simulink model "MicroMouseDebug"  (R2023a)
settings: Solver=VariableStepAuto  StartTime=0.0  StopTime=inf  FixedStep=0.001  RelTol=1e-3
model workspace (MAT data in the model file):
  comPort = "COM6"
  numBytes = Simulink.Parameter
  numBytes.Value = 5
  numBytes.DataType = 'auto'
  numBytes.Complexity = 'real'
  numBytes.Dimensions = [1 1]
libraries: etargetslib x37, dspstat3 x34, instrumentseriallib x2, stmutilitieslib x1
settings Model: Creator=JesseJabezArendse  LastModifiedBy=JesseJabezArendse
settings DataIOCC: SaveOutput=off  SaveTime=off
settings OptimizationCC: DefaultParameterBehavior=Inlined  InlineInvariantSignals=on  EnhancedBackFolding=on  PassReuseOutputArgsAs=Individual arguments  StateBitsets=on  DataBitsets=on  ZeroExternalMemoryAtStartup=off  ZeroInternalMemoryAtStartup=off  NoFixptDivByZeroProtection=on  EfficientFloat2IntCast=on  OptimizeBlockOrder=speed  DifferentSizesBufferReuse=on  EfficientTunableParamExpr=on
settings DebuggingCC: ParameterPrecisionLossMsg=none  ParameterTunabilityLossMsg=error
settings SFSimCC: MATLABDynamicMemAlloc=off
settings RTWCC: Description=Embedded Coder  SystemTargetFile=ert.tlc  TemplateMakefile=ert_default_tmf  GenerateReport=on  RTWVerbose=off  IncludeHyperlinkInReport=on  LaunchReport=on  GenerateTraceInfo=on  GenerateTraceReport=on  GenerateTraceReportSl=on  GenerateTraceReportSf=on  GenerateTraceReportEml=on
settings CodeAppCC: ForceParamTrailComments=on  IgnoreCustomStorageClasses=off  OperatorAnnotations=on  SimulinkDataObjDesc=on  SFDataObjDesc=on  CustomSymbolStrGlobalVar=rt$N$M  CustomSymbolStrType=$N$M  CustomSymbolStrFcn=$N$M$F  CustomSymbolStrMacro=$N$M  InsertBlockDesc=on
settings ERTTargetCC: TargetLangStandard=C99 (ISO)  GenerateSampleERTMain=on  IncludeMdlTerminateFcn=off  CombineSignalStateStructs=on  PurelyIntegerCode=on  SupportNonFinite=off  InlinedParameterPlacement=NonHierarchical  ERTCustomFileTemplate=example_file_process.tlc

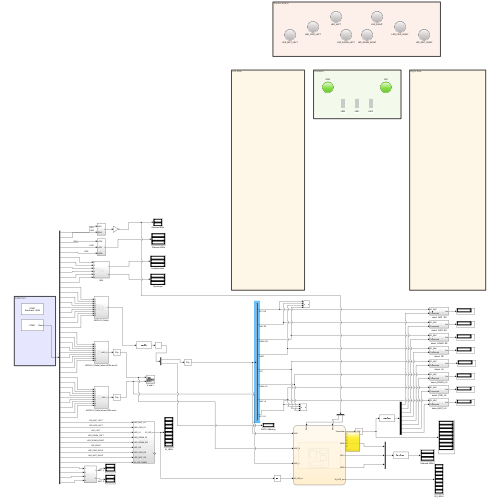
[thumbnail: Simulink's stored preview of the top-level diagram]
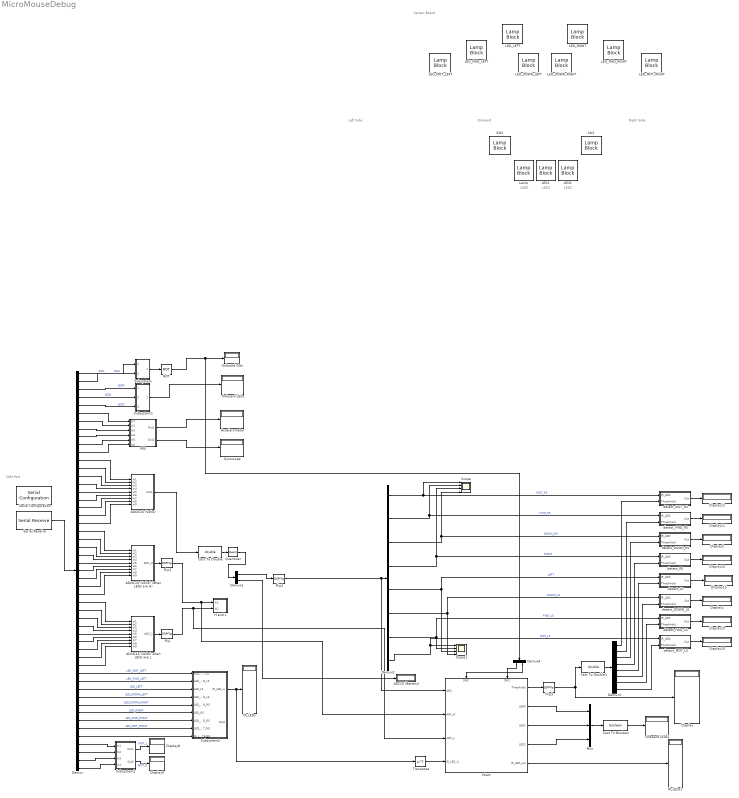
== system MicroMouseDebug ==
  note: Onboard
  note: LED0
  note: LED1
  note: LED2
  note: Left Side
  note: COM Port
  note: Right Side
  note: Sensor Board
  ADC16 (Battery) : Display
  ADC8-16 (Volts) : Subsystem
  ADC8-16 (Volts) (when LEDs are H) : Subsystem
  ADC8-16 (Volts) when LEDs are L : Subsystem
  Accelerometer : Display
  Cast To Boolean : DataTypeConversion  OutDataTypeStr=boolean  SaturateOnIntegerOverflow=off  RndMeth=Floor
  Cast To Double : DataTypeConversion  OutDataTypeStr=double  SaturateOnIntegerOverflow=off  RndMeth=Floor
  Cast To Double1 : DataTypeConversion  OutDataTypeStr=double  SaturateOnIntegerOverflow=off  RndMeth=Floor
  Chart : Stateflow chart  TreatAsAtomicUnit=on
      settings: PortSchema="{\"entries\":[{\"content\":{\"sides\":[{\"content\":{\"connectorIds\":[\"In1\",\"In4\",\"In5\",\"In6\"]},\"type\":\"ConnectorPlacement.EquallySpacedRectSide\",\"uuid\":\"32f6fed0-3232-4bab-b39d-a3af84b75639\"},{\"content\":{\"connectorIds\":[\"Out5\",\"Out1\",\"Out2\",\"Out3\",\"Out4\"],\"side\":\"RIGHT\"},\"type\":\"ConnectorPlacement.EquallySpacedRectSide\",\"uuid\":\"0c32a1fe-915a-4e8a-b3ee-800457e23572\"},{\"content\":{\"connectorIds\":[\"In3\",\"In2\"],\"side\":\"TOP\"},\"type\":\"ConnectorPlacement.EquallySpacedRectSide\",\"uuid\":\"1ac04b60-bb97-4700-a588-8796c93b1b04\"}]},\"type\":\"ConnectorPlacement.EquallySpacedConnector\",\"uuid\":\"e2f36b59-a9e2-4f43-a02a-04bcc2f7ebe2\"}],\"packageUris\":[\"http://schema.mathworks.com/mf0/Connector/R2020b\"],\"version\":\"1.0\"}"
  Demux : Demux  Outputs=[1 1 1 1 1 4 4 4 4 4 4 2 2 2 2 2 2 2 2 2 2 2 2 2 2 2 2 2 2 2 2 2 2 2 2 2 2 2 1 1 1 1 1 1 1 1 4 2 2 2 2]
  Demux1 : Demux  Outputs=[8 1]
  Demux2 : Demux  Outputs=8
  Demux3 : Demux  Outputs=8
  Demux4 : Demux  Outputs=2
  Display{,1..2,8..15} (11 alike) : Display
  Flip{,1..3} (4 alike) : DSPFlip
  Gyroscope : Display
  H and L : Subsystem
  IMU : Subsystem
  IR_LEDs : Display
  IR_LEDs1 : Display
  LED1 : LampBlock  LabelPosition=Hide  Icon=Rectangle
  LED2 : LampBlock  LabelPosition=Hide  Icon=Rectangle
  LED_DOWN_LEFT : LampBlock  LabelPosition=Hide
  LED_DOWN_RIGHT : LampBlock  LabelPosition=Hide
  LED_FWD_LEFT : LampBlock  LabelPosition=Hide
  LED_FWD_RIGHT : LampBlock  LabelPosition=Hide
  LED_LEFT : LampBlock  LabelPosition=Hide
  LED_MOT_LEFT : LampBlock  LabelPosition=Hide
  LED_MOT_RIGHT : LampBlock  LabelPosition=Hide
  LED_RIGHT : LampBlock  LabelPosition=Hide
  Lamp : LampBlock  LabelPosition=Hide  Icon=Rectangle
  Mux : Mux  Inputs=3
  NOT : Logic  Operator=NOT  IconShape=distinctive  AllPortsSameDT=off  OutDataTypeStr=boolean
  Onboard LEDs : Display
  Onboard LEDs1 : Display
  Onboard SWs : Display
  Quantizer : Quantizer  QuantizationInterval=0.01
  SW1 : LampBlock  LabelPosition=Hide
  SW2 : LampBlock  LabelPosition=Hide
  Scope : Scope  NumInputPorts=4
  Scope1 : Scope  NumInputPorts=4
  Serial Configuration : instrumentseriallib/Serial Configuration  Priority=-200000  PortSel=COM7  Port=COM7  ComPort=COM7  BaudRate=9600  DataBits=8  Parity=none  StopBits=1  ByteOrder=little-endian  FlowControl=none  Timeout=10  SimulateUsing=Interpreted execution  BlockInModel=on  aMode=1
      settings: LibrarySourceBlock=embeddedtargetslib/Host Communication/Serial Configuration
  Serial Receive : instrumentseriallib/Serial Receive  Priority=1  PortSel=COM7  Port=COM7  ComPort=COM7  DataType=uint8  SaveDataType=uint8  ToggleHeader=on  Header='JJA'  ToggleTerminator=on  Terminator=Custom terminator  CustomTerminator='3099'  InputFormat=Column major  ToggleDataSize=on  DataSize=[1 103]  EnableBlockingMode=on  ActionDataUnavailable=Output last received value  ActionWhenDataUnavailable=Output last received value  CustomValue=0  SampleTime=0.01  SimulateUsing=Interpreted execution  BlockInModel=on  aMode=1
      settings: LibrarySourceBlock=embeddedtargetslib/Host Communication/Serial Receive
  Subsystem : Subsystem
  Subsystem1 : Subsystem
  Subsystem2 : Subsystem
  Subsystem3 : Subsystem
  Transpose : Math  Operator=transpose
  detect_DOWN_LS : Subsystem
  detect_DOWN_RS : Subsystem
  detect_FWD_LS : Subsystem
  detect_FWD_RS : Subsystem
  detect_LS : Subsystem
  detect_MOT_LS : Subsystem
  detect_MOT_RS : Subsystem
  detect_RS : Subsystem
  wires:
  Serial Receive/1 -> Demux/1
  Demux1/2 -> ADC16 (Battery)/1
  Demux/12 -> ADC8-16 (Volts)/1(In1)
  Demux/13 -> ADC8-16 (Volts)/2(In2)
  Demux/14 -> ADC8-16 (Volts)/3(In3)
  Demux/15 -> ADC8-16 (Volts)/4(In4)
  Demux/16 -> ADC8-16 (Volts)/5(In5)
  Demux/17 -> ADC8-16 (Volts)/6(In6)
  Demux/18 -> ADC8-16 (Volts)/7(In7)
  Demux/19 -> ADC8-16 (Volts)/8(In8)
  Demux/20 -> ADC8-16 (Volts)/9(In9)
  Demux/6 -> IMU/1(In1)
  Demux/7 -> IMU/2(In2)
  Demux/8 -> IMU/3(In3)
  Demux/9 -> IMU/4(In4)
  Demux/10 -> IMU/5(In5)
  Demux/11 -> IMU/6(In6)
  IMU/1(Out1) -> Accelerometer/1
  IMU/2(Out2) -> Gyroscope/1
  Demux/1 -> Subsystem/1(SW1)  "SW1"
  Demux/2 -> Subsystem/2(SW2)  "SW2"
  Subsystem/1(Out1) -> NOT/1
  Demux/3 -> Subsystem1/1(LED0)  "LED0"
  Demux/4 -> Subsystem1/2(LED1)  "LED1"
  Demux/5 -> Subsystem1/3(LED2)  "LED2"
  Subsystem1/1(Out1) -> Onboard LEDs/1
  Demux/38 -> ADC8-16 (Volts) when LEDs are L/9(In9)
  Demux/37 -> ADC8-16 (Volts) when LEDs are L/8(In8)
  Demux/34 -> ADC8-16 (Volts) when LEDs are L/5(In5)
  Demux/33 -> ADC8-16 (Volts) when LEDs are L/4(In4)
  Demux/35 -> ADC8-16 (Volts) when LEDs are L/6(In6)
  Demux/32 -> ADC8-16 (Volts) when LEDs are L/3(In3)
  Demux/36 -> ADC8-16 (Volts) when LEDs are L/7(In7)
  Demux/31 -> ADC8-16 (Volts) when LEDs are L/2(In2)
  Demux/30 -> ADC8-16 (Volts) when LEDs are L/1(In1)
  Demux/29 -> ADC8-16 (Volts) (when LEDs are H)/9(In9)
  Demux/28 -> ADC8-16 (Volts) (when LEDs are H)/8(In8)
  Demux/25 -> ADC8-16 (Volts) (when LEDs are H)/5(In5)
  Demux/24 -> ADC8-16 (Volts) (when LEDs are H)/4(In4)
  Demux/26 -> ADC8-16 (Volts) (when LEDs are H)/6(In6)
  Demux/23 -> ADC8-16 (Volts) (when LEDs are H)/3(In3)
  Demux/27 -> ADC8-16 (Volts) (when LEDs are H)/7(In7)
  Demux/22 -> ADC8-16 (Volts) (when LEDs are H)/2(In2)
  Demux/21 -> ADC8-16 (Volts) (when LEDs are H)/1(In1)
  Demux/39 -> Subsystem3/1(LED_MOT_LS)  "LED_MOT_LEFT"
  Demux/40 -> Subsystem3/2(LED_FWD_LS)  "LED_FWD_LEFT"
  Demux/41 -> Subsystem3/3(LED_LS)  "LED_LEFT"
  Demux/46 -> Subsystem3/8(LED_MOT_RS)  "LED_MOT_RIGHT"
  Demux/47 -> Subsystem3/9(IR_LED_TIMER)
  ADC8-16 (Volts)/1(Out1) -> Cast To Double/1
  detect_FWD_LS/1(Out) -> Display13/1
  Cast To Double/1 -> Quantizer/1
  detect_MOT_LS/1(Out) -> Display10/1
  detect_FWD_RS/1(Out) -> Display11/1
  detect_MOT_RS/1(Out) -> Display12/1
  detect_RS/1(Out) -> Display14/1
  detect_LS/1(Out) -> Display15/1
  Subsystem2/2(Out2) -> Display9/1  "MOT_R"
  Demux/50 -> Subsystem2/3(In3)
  Demux/48 -> Subsystem2/1(In1)
  Demux/51 -> Subsystem2/4(In4)
  Subsystem2/1(Out1) -> Display8/1  "MOT_L"
  Demux/49 -> Subsystem2/2(In2)
  Demux/42 -> Subsystem3/4(LED_DOWN_LS)  "LED_DOWN_LEFT"
  Demux/43 -> Subsystem3/5(LED_DOWN_RS)  "LED_DOWN_RIGHT"
  Demux/44 -> Subsystem3/6(LED_RS)  "LED_RIGHT"
  Demux/45 -> Subsystem3/7(LED_FWD_RS)  "LED_FWD_RIGHT"
  Demux2/1 -> detect_MOT_RS/1(IR_ADC), Scope/1  "MOT_RS"
  Demux2/2 -> Scope/2, detect_FWD_RS/1(IR_ADC)  "FWD_RS"
  Demux2/3 -> Scope/4, detect_DOWN_RS/1(IR_ADC)  "DOWN_RS"
  Demux2/4 -> Scope/3, detect_RS/1(IR_ADC)  "RIGHT"
  Demux2/5 -> detect_LS/1(IR_ADC), Scope1/3  "LEFT"
  Demux2/6 -> detect_DOWN_LS/1(IR_ADC), Scope1/4  "DOWN_LS"
  Demux2/7 -> detect_FWD_LS/1(IR_ADC), Scope1/2  "FWD_LS"
  Demux2/8 -> detect_MOT_LS/1(IR_ADC), Scope1/1  "MOT_LS"
  detect_DOWN_LS/1(Out) -> Display1/1
  detect_DOWN_RS/1(Out) -> Display2/1
  Quantizer/1 -> Demux1/1
  Subsystem3/1(IR_LED_in) -> Transpose/1, IR_LEDs/1
  Chart/1(LED0) -> Mux/1
  Chart/2(LED1) -> Mux/2
  Chart/3(LED2) -> Mux/3
  Mux/1 -> Cast To Boolean/1
  Demux1/1 -> Flip2/1
  ADC8-16 (Volts) (when LEDs are H)/1(ADC_H) -> Flip1/1
  ADC8-16 (Volts) when LEDs are L/1(ADC_L) -> Flip/1
  Chart/4(IR_LED_out) -> IR_LEDs1/1
  Chart/5(Thresholds) -> Flip3/1
  Flip/1 -> Chart/5(ADC_L), H and L/2(In2)
  Flip1/1 -> Chart/4(ADC_H), H and L/1(In1)
  Flip2/1 -> Chart/1(ADC), Demux2/1
  Demux3/1 -> detect_MOT_RS/2(Threshhold)
  Demux3/2 -> detect_FWD_RS/2(Threshhold)
  Demux3/3 -> detect_DOWN_RS/2(Threshhold)
  Demux3/4 -> detect_RS/2(Threshhold)
  Demux3/5 -> detect_LS/2(Threshhold)
  Demux3/6 -> detect_DOWN_LS/2(Threshhold)
  Demux3/7 -> detect_FWD_LS/2(Threshhold)
  Demux3/8 -> detect_MOT_LS/2(Threshhold)
  Demux4/1 -> Chart/2(SW1)
  Demux4/2 -> Chart/3(SW2)
  Transpose/1 -> Chart/6(IR_LED_in)
  Cast To Boolean/1 -> Onboard LEDs1/1
  Cast To Double1/1 -> Demux3/1
  NOT/1 -> Demux4/1, Onboard SWs/1
  Flip3/1 -> Display/1, Cast To Double1/1

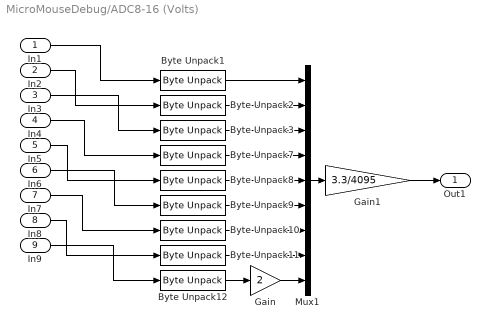
== system MicroMouseDebug/ADC8-16 (Volts) ==
  In1 : Inport
  In2 : Inport  Port=2
  In3 : Inport  Port=3
  In4 : Inport  Port=4
  In5 : Inport  Port=5
  In6 : Inport  Port=6
  In7 : Inport  Port=7
  In8 : Inport  Port=8
  In9 : Inport  Port=9
  Byte Unpack{1..3,7..12} (9 alike) : etargetslib/Byte Unpack  dimensions={[1]}  datatypes={'uint16'}  byteAlign=1
  Gain : Gain  Gain=2  OutDataTypeStr=uint16
  Gain1 : Gain  Gain=3.3/4095
  Mux1 : Mux  Inputs=9
  Out1 : Outport
  wires:
  In7/1 -> Byte Unpack10/1
  Byte Unpack11/1 -> Mux1/8
  Byte Unpack8/1 -> Mux1/5
  Byte Unpack2/1 -> Mux1/2
  Byte Unpack12/1 -> Gain/1
  Byte Unpack7/1 -> Mux1/4
  In4/1 -> Byte Unpack7/1
  Byte Unpack1/1 -> Mux1/1
  In1/1 -> Byte Unpack1/1
  Gain/1 -> Mux1/9
  In6/1 -> Byte Unpack9/1
  Byte Unpack10/1 -> Mux1/7
  Byte Unpack9/1 -> Mux1/6
  Byte Unpack3/1 -> Mux1/3
  Mux1/1 -> Gain1/1
  Gain1/1 -> Out1/1
  In8/1 -> Byte Unpack11/1
  In3/1 -> Byte Unpack3/1
  In5/1 -> Byte Unpack8/1
  In2/1 -> Byte Unpack2/1
  In9/1 -> Byte Unpack12/1

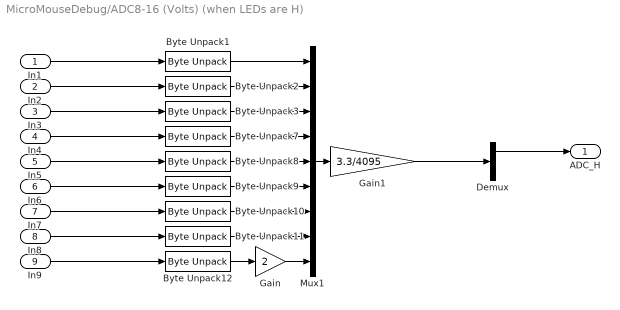
== system MicroMouseDebug/ADC8-16 (Volts) (when LEDs are H) ==
  In1 : Inport
  In2 : Inport  Port=2
  In3 : Inport  Port=3
  In4 : Inport  Port=4
  In5 : Inport  Port=5
  In6 : Inport  Port=6
  In7 : Inport  Port=7
  In8 : Inport  Port=8
  In9 : Inport  Port=9
  Byte Unpack{1..3,7..12} (9 alike) : etargetslib/Byte Unpack  dimensions={[1]}  datatypes={'uint16'}  byteAlign=1
  Demux : Demux  Outputs=[8 1]
  Gain : Gain  Gain=2  OutDataTypeStr=uint16
  Gain1 : Gain  Gain=3.3/4095
  Mux1 : Mux  Inputs=9
  ADC_H : Outport
  wires:
  In7/1 -> Byte Unpack10/1
  Byte Unpack11/1 -> Mux1/8
  Byte Unpack8/1 -> Mux1/5
  Byte Unpack2/1 -> Mux1/2
  Byte Unpack12/1 -> Gain/1
  Byte Unpack7/1 -> Mux1/4
  In4/1 -> Byte Unpack7/1
  Byte Unpack1/1 -> Mux1/1
  In1/1 -> Byte Unpack1/1
  Gain/1 -> Mux1/9
  In6/1 -> Byte Unpack9/1
  Byte Unpack10/1 -> Mux1/7
  Byte Unpack9/1 -> Mux1/6
  Byte Unpack3/1 -> Mux1/3
  Mux1/1 -> Gain1/1
  Gain1/1 -> Demux/1
  In8/1 -> Byte Unpack11/1
  In3/1 -> Byte Unpack3/1
  In5/1 -> Byte Unpack8/1
  In2/1 -> Byte Unpack2/1
  In9/1 -> Byte Unpack12/1
  Demux/1 -> ADC_H/1

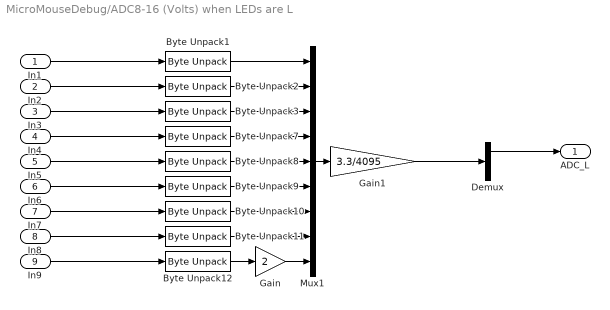
== system MicroMouseDebug/ADC8-16 (Volts) when LEDs are L ==
  In1 : Inport
  In2 : Inport  Port=2
  In3 : Inport  Port=3
  In4 : Inport  Port=4
  In5 : Inport  Port=5
  In6 : Inport  Port=6
  In7 : Inport  Port=7
  In8 : Inport  Port=8
  In9 : Inport  Port=9
  Byte Unpack{1..3,7..12} (9 alike) : etargetslib/Byte Unpack  dimensions={[1]}  datatypes={'uint16'}  byteAlign=1
  Demux : Demux  Outputs=[8 1]
  Gain : Gain  Gain=2  OutDataTypeStr=uint16
  Gain1 : Gain  Gain=3.3/4095
  Mux1 : Mux  Inputs=9
  ADC_L : Outport
  wires:
  In7/1 -> Byte Unpack10/1
  Byte Unpack11/1 -> Mux1/8
  Byte Unpack8/1 -> Mux1/5
  Byte Unpack2/1 -> Mux1/2
  Byte Unpack12/1 -> Gain/1
  Byte Unpack7/1 -> Mux1/4
  In4/1 -> Byte Unpack7/1
  Byte Unpack1/1 -> Mux1/1
  In1/1 -> Byte Unpack1/1
  Gain/1 -> Mux1/9
  In6/1 -> Byte Unpack9/1
  Byte Unpack10/1 -> Mux1/7
  Byte Unpack9/1 -> Mux1/6
  Byte Unpack3/1 -> Mux1/3
  Mux1/1 -> Gain1/1
  In8/1 -> Byte Unpack11/1
  In3/1 -> Byte Unpack3/1
  In5/1 -> Byte Unpack8/1
  In2/1 -> Byte Unpack2/1
  In9/1 -> Byte Unpack12/1
  Gain1/1 -> Demux/1
  Demux/1 -> ADC_L/1

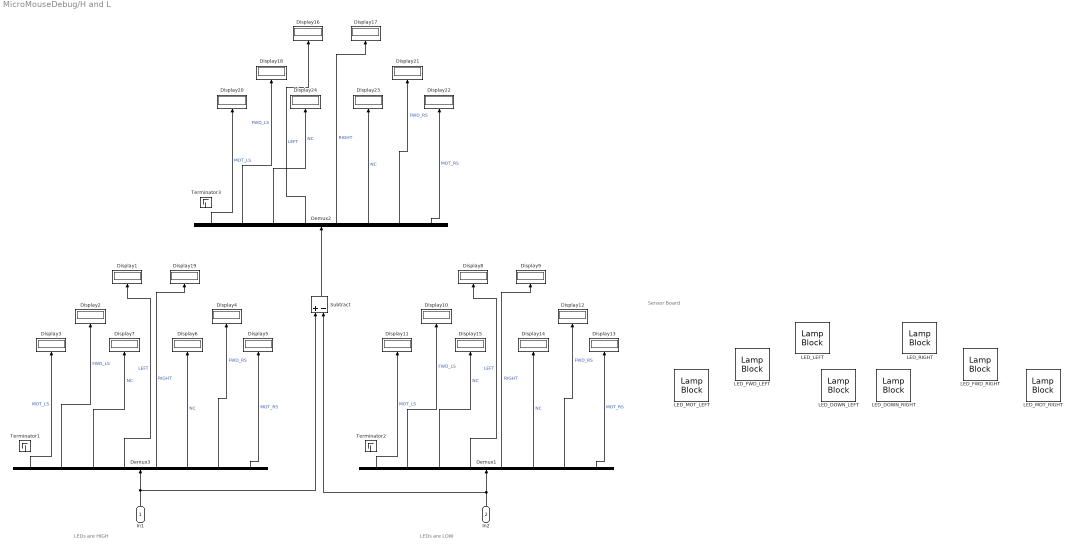
== system MicroMouseDebug/H and L ==
  note: LEDs are HIGH
  note: Sensor Board
  note: LEDs are LOW
  In1 : Inport
  In2 : Inport  Port=2
  Demux1 : Demux  Outputs=8
  Demux2 : Demux  Outputs=8
  Demux3 : Demux  Outputs=8
  Display{1..24} (24 alike) : Display
      settings: Decimation=2
  LED_DOWN_LEFT : LampBlock  LabelPosition=Hide
  LED_DOWN_RIGHT : LampBlock  LabelPosition=Hide
  LED_FWD_LEFT : LampBlock  LabelPosition=Hide
  LED_FWD_RIGHT : LampBlock  LabelPosition=Hide
  LED_LEFT : LampBlock  LabelPosition=Hide
  LED_MOT_LEFT : LampBlock  LabelPosition=Hide
  LED_MOT_RIGHT : LampBlock  LabelPosition=Hide
  LED_RIGHT : LampBlock  LabelPosition=Hide
  Subtract : Sum  Inputs=+-  AccumDataTypeStr=double  OutDataTypeStr=Inherit: Same as accumulator  RndMeth=Nearest  SaturateOnIntegerOverflow=on
  Terminator1 : Terminator
  Terminator2 : Terminator
  Terminator3 : Terminator
  wires:
  Demux3/5 -> Display1/1  "LEFT"
  Demux3/2 -> Display4/1  "FWD_RS"
  Demux3/7 -> Display2/1  "FWD_LS"
  Demux3/4 -> Display19/1  "RIGHT"
  Demux3/8 -> Display3/1  "MOT_LS"
  Demux3/3 -> Display6/1  "NC"
  Demux3/6 -> Display7/1  "NC"
  Demux3/1 -> Display5/1  "MOT_RS"
  ? -> Terminator1/1
  In1/1 -> Demux3/1, Subtract/1
  Demux1/2 -> Display12/1  "FWD_RS"
  In2/1 -> Demux1/1, Subtract/2
  Demux1/1 -> Display13/1  "MOT_RS"
  Demux1/3 -> Display14/1  "NC"
  Demux1/5 -> Display8/1  "LEFT"
  Demux1/8 -> Display11/1  "MOT_LS"
  Demux1/4 -> Display9/1  "RIGHT"
  Demux1/6 -> Display15/1  "NC"
  ? -> Terminator2/1
  Demux1/7 -> Display10/1  "FWD_LS"
  Demux2/2 -> Display21/1  "FWD_RS"
  Demux2/1 -> Display22/1  "MOT_RS"
  Demux2/3 -> Display23/1  "NC"
  Demux2/5 -> Display16/1  "LEFT"
  Demux2/8 -> Display20/1  "MOT_LS"
  Demux2/4 -> Display17/1  "RIGHT"
  Demux2/6 -> Display24/1  "NC"
  ? -> Terminator3/1
  Demux2/7 -> Display18/1  "FWD_LS"
  Subtract/1 -> Demux2/1

== system MicroMouseDebug/IMU ==
  In1 : Inport
  In2 : Inport  Port=2
  In3 : Inport  Port=3
  In4 : Inport  Port=4
  In5 : Inport  Port=5
  In6 : Inport  Port=6
  Byte Unpack{4..6,13..15} (6 alike) : etargetslib/Byte Unpack  dimensions={[1]}  datatypes={'single'}  byteAlign=1
  Mux : Mux  Inputs=3
  Mux2 : Mux  Inputs=3
  Out1 : Outport
  Out2 : Outport  Port=2
  wires:
  Byte Unpack4/1 -> Mux/1
  Byte Unpack14/1 -> Mux2/2
  Byte Unpack15/1 -> Mux2/3
  Mux2/1 -> Out2/1
  Byte Unpack13/1 -> Mux2/1
  In6/1 -> Byte Unpack15/1
  In3/1 -> Byte Unpack6/1
  Byte Unpack5/1 -> Mux/2
  Byte Unpack6/1 -> Mux/3
  In4/1 -> Byte Unpack13/1
  In1/1 -> Byte Unpack4/1
  In2/1 -> Byte Unpack5/1
  Mux/1 -> Out1/1
  In5/1 -> Byte Unpack14/1

== system MicroMouseDebug/Subsystem ==
  SW1 : Inport
  SW2 : Inport  Port=2
  Mux4 : Mux  Inputs=2
  Out1 : Outport
  wires:
  Mux4/1 -> Out1/1
  SW2/1 -> Mux4/2
  SW1/1 -> Mux4/1

== system MicroMouseDebug/Subsystem1 ==
  LED0 : Inport
  LED1 : Inport  Port=2
  LED2 : Inport  Port=3
  Mux3 : Mux  Inputs=3
  Out1 : Outport
  wires:
  Mux3/1 -> Out1/1
  LED2/1 -> Mux3/3
  LED0/1 -> Mux3/1
  LED1/1 -> Mux3/2

== system MicroMouseDebug/Subsystem2 ==
  In1 : Inport
  In2 : Inport  Port=2
  In3 : Inport  Port=3
  In4 : Inport  Port=4
  Byte Unpack{1..3,7} (4 alike) : etargetslib/Byte Unpack  dimensions={[1]}  datatypes={'uint16'}  byteAlign=1
  Gain : Gain  Gain=100/1600
  Gain1 : Gain  Gain=100/1600
  Mux1 : Mux  Inputs=2
  Mux2 : Mux  Inputs=2
  Out1 : Outport
  Out2 : Outport  Port=2
  wires:
  Byte Unpack2/1 -> Mux1/2  "MOT_L_BWD"
  In1/1 -> Byte Unpack1/1
  Byte Unpack3/1 -> Mux2/1  "MOT_R_FWD"
  Mux2/1 -> Gain1/1
  Byte Unpack7/1 -> Mux2/2  "MOT_R_BWD"
  Mux1/1 -> Gain/1
  Gain/1 -> Out1/1
  Byte Unpack1/1 -> Mux1/1  "MOT_L_FWD"
  In3/1 -> Byte Unpack3/1
  In2/1 -> Byte Unpack2/1
  In4/1 -> Byte Unpack7/1
  Gain1/1 -> Out2/1

== system MicroMouseDebug/Subsystem3 ==
  LED_MOT_LS : Inport
  LED_FWD_LS : Inport  Port=2
  LED_LS : Inport  Port=3
  LED_DOWN_LS : Inport  Port=4
  LED_DOWN_RS : Inport  Port=5
  LED_RS : Inport  Port=6
  LED_FWD_RS : Inport  Port=7
  LED_MOT_RS : Inport  Port=8
  IR_LED_TIMER : Inport  Port=9
  Byte Unpack : stmutilitieslib/Byte Unpack  dimensions={[1]}  datatypes={'uint32'}  byteAlign=1  blockPlatform=stm32f4discovery
  Mux : Mux  Inputs=8
  IR_LED_in : Outport
  Out2 : Outport  Port=2
  wires:
  IR_LED_TIMER/1 -> Byte Unpack/1
  Mux/1 -> IR_LED_in/1
  LED_FWD_LS/1 -> Mux/2
  LED_LS/1 -> Mux/3
  LED_MOT_LS/1 -> Mux/1
  Byte Unpack/1 -> Out2/1
  LED_FWD_RS/1 -> Mux/7
  LED_MOT_RS/1 -> Mux/8
  LED_RS/1 -> Mux/6
  LED_DOWN_LS/1 -> Mux/4
  LED_DOWN_RS/1 -> Mux/5

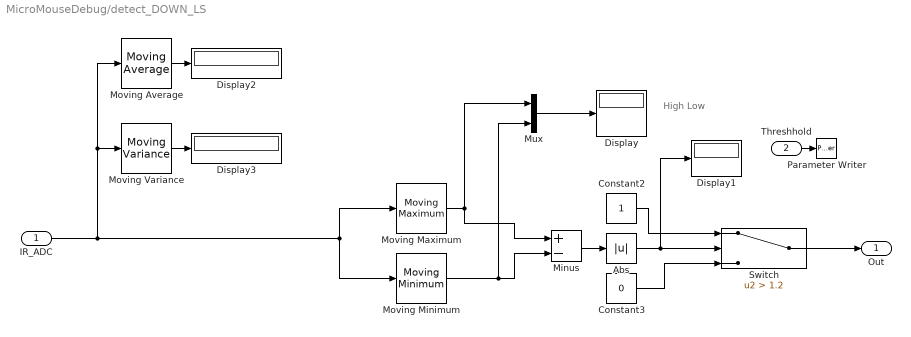
== system MicroMouseDebug/detect_DOWN_LS ==
  note: High
      | Low
  IR_ADC : Inport
  Threshhold : Inport  Port=2
  Abs : Abs  SaturateOnIntegerOverflow=off
  Constant2 : Constant
  Constant3 : Constant  Value=0
  Display{,1..3} (4 alike) : Display
  Minus : Sum  Inputs=+-  AccumDataTypeStr=single  OutDataTypeStr=single
  Moving Average : dspstat3/Moving Average  Method=Sliding window  ForgettingFactorPort=off  SpecifyWindowLength=on  WindowLength=4  OverlapLength=3  AllowArbitraryInputLength=off  ForgettingFactor=0.9  SimulateUsing=Code generation
  Moving Maximum : dspstat3/Moving Maximum  SpecifyWindowLength=on  WindowLength=15  SimulateUsing=Code generation
  Moving Minimum : dspstat3/Moving Minimum  SpecifyWindowLength=on  WindowLength=15  SimulateUsing=Code generation
  Moving Variance : dspstat3/Moving Variance  Method=Sliding window  ForgettingFactorPort=off  SpecifyWindowLength=on  WindowLength=4  OverlapLength=3  AllowArbitraryInputLength=off  ForgettingFactor=0.9  SimulateUsing=Code generation
  Mux : Mux  Inputs=2
  Parameter Writer : ParameterWriter  ParameterOwnerBlock=../Switch  ParameterName=Threshold  ParameterInternalName=Threshold
  Switch : Switch  Criteria=u2 > Threshold  Threshold=1.2  SaturateOnIntegerOverflow=off  InputSameDT=off
  Out : Outport
  wires:
  Minus/1 -> Abs/1
  Constant2/1 -> Switch/1
  Moving Minimum/1 -> Mux/2, Minus/2
  Switch/1 -> Out/1
  Constant3/1 -> Switch/3
  Moving Maximum/1 -> Mux/1, Minus/1
  Mux/1 -> Display/1
  IR_ADC/1 -> Moving Average/1, Moving Variance/1, Moving Minimum/1, Moving Maximum/1
  Abs/1 -> Switch/2, Display1/1
  Moving Average/1 -> Display2/1
  Moving Variance/1 -> Display3/1
  Threshhold/1 -> Parameter Writer/1

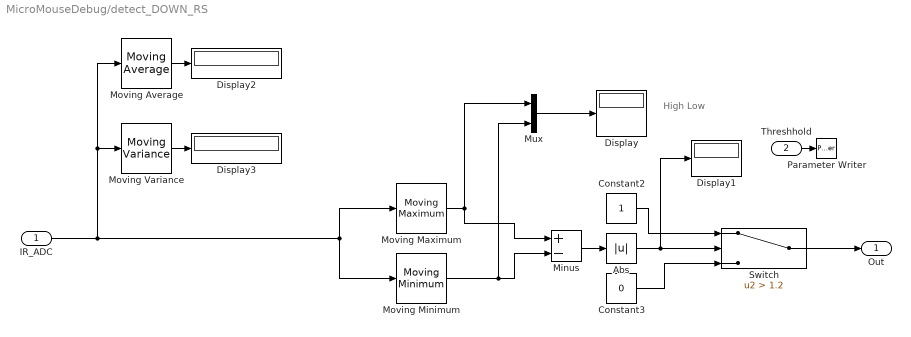
== system MicroMouseDebug/detect_DOWN_RS ==
  note: High
      | Low
  IR_ADC : Inport
  Threshhold : Inport  Port=2
  Abs : Abs  SaturateOnIntegerOverflow=off
  Constant2 : Constant
  Constant3 : Constant  Value=0
  Display{,1..3} (4 alike) : Display
  Minus : Sum  Inputs=+-  AccumDataTypeStr=single  OutDataTypeStr=single
  Moving Average : dspstat3/Moving Average  Method=Sliding window  ForgettingFactorPort=off  SpecifyWindowLength=on  WindowLength=4  OverlapLength=3  AllowArbitraryInputLength=off  ForgettingFactor=0.9  SimulateUsing=Code generation
  Moving Maximum : dspstat3/Moving Maximum  SpecifyWindowLength=on  WindowLength=15  SimulateUsing=Code generation
  Moving Minimum : dspstat3/Moving Minimum  SpecifyWindowLength=on  WindowLength=15  SimulateUsing=Code generation
  Moving Variance : dspstat3/Moving Variance  Method=Sliding window  ForgettingFactorPort=off  SpecifyWindowLength=on  WindowLength=4  OverlapLength=3  AllowArbitraryInputLength=off  ForgettingFactor=0.9  SimulateUsing=Code generation
  Mux : Mux  Inputs=2
  Parameter Writer : ParameterWriter  ParameterOwnerBlock=../Switch  ParameterName=Threshold  ParameterInternalName=Threshold
  Switch : Switch  Criteria=u2 > Threshold  Threshold=1.2  SaturateOnIntegerOverflow=off  InputSameDT=off
  Out : Outport
  wires:
  Minus/1 -> Abs/1
  Constant2/1 -> Switch/1
  Moving Minimum/1 -> Mux/2, Minus/2
  Switch/1 -> Out/1
  Constant3/1 -> Switch/3
  Moving Maximum/1 -> Mux/1, Minus/1
  Mux/1 -> Display/1
  IR_ADC/1 -> Moving Average/1, Moving Variance/1, Moving Minimum/1, Moving Maximum/1
  Abs/1 -> Switch/2, Display1/1
  Moving Average/1 -> Display2/1
  Moving Variance/1 -> Display3/1
  Threshhold/1 -> Parameter Writer/1

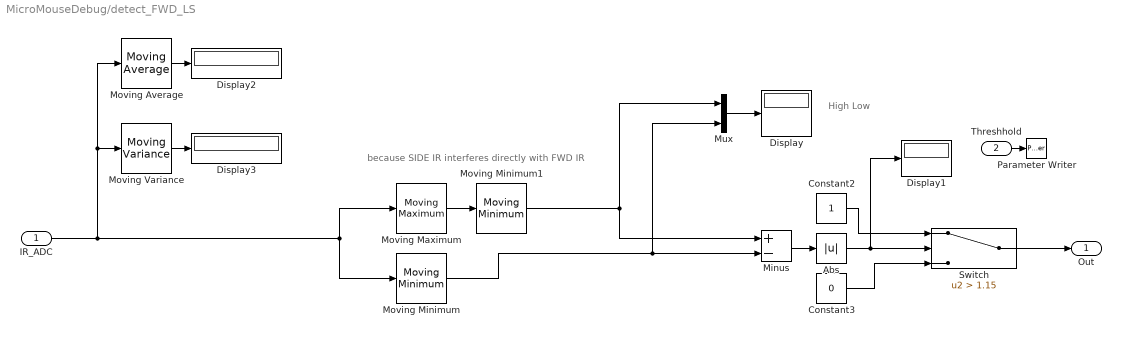
== system MicroMouseDebug/detect_FWD_LS ==
  note: because SIDE IR interferes directly with FWD IR
  note: High
      | Low
  IR_ADC : Inport
  Threshhold : Inport  Port=2
  Abs : Abs  SaturateOnIntegerOverflow=off
  Constant2 : Constant
  Constant3 : Constant  Value=0
  Display{,1..3} (4 alike) : Display
  Minus : Sum  Inputs=+-  AccumDataTypeStr=single  OutDataTypeStr=single
  Moving Average : dspstat3/Moving Average  Method=Sliding window  ForgettingFactorPort=off  SpecifyWindowLength=on  WindowLength=4  OverlapLength=3  AllowArbitraryInputLength=off  ForgettingFactor=0.9  SimulateUsing=Code generation
  Moving Maximum : dspstat3/Moving Maximum  SpecifyWindowLength=on  WindowLength=5  SimulateUsing=Code generation
  Moving Minimum : dspstat3/Moving Minimum  SpecifyWindowLength=on  WindowLength=15  SimulateUsing=Code generation
  Moving Minimum1 : dspstat3/Moving Minimum  SpecifyWindowLength=on  WindowLength=15  SimulateUsing=Code generation
  Moving Variance : dspstat3/Moving Variance  Method=Sliding window  ForgettingFactorPort=off  SpecifyWindowLength=on  WindowLength=4  OverlapLength=3  AllowArbitraryInputLength=off  ForgettingFactor=0.9  SimulateUsing=Code generation
  Mux : Mux  Inputs=2
  Parameter Writer : ParameterWriter  ParameterOwnerBlock=../Switch  ParameterName=Threshold  ParameterInternalName=Threshold
  Switch : Switch  Criteria=u2 > Threshold  Threshold=1.15  SaturateOnIntegerOverflow=off  InputSameDT=off
  Out : Outport
  wires:
  Moving Maximum/1 -> Moving Minimum1/1
  Moving Minimum1/1 -> Mux/1, Minus/1
  IR_ADC/1 -> Moving Average/1, Moving Variance/1, Moving Minimum/1, Moving Maximum/1
  Abs/1 -> Switch/2, Display1/1
  Moving Variance/1 -> Display3/1
  Moving Average/1 -> Display2/1
  Switch/1 -> Out/1
  Constant3/1 -> Switch/3
  Constant2/1 -> Switch/1
  Mux/1 -> Display/1
  Minus/1 -> Abs/1
  Threshhold/1 -> Parameter Writer/1
  Moving Minimum/1 -> Minus/2, Mux/2

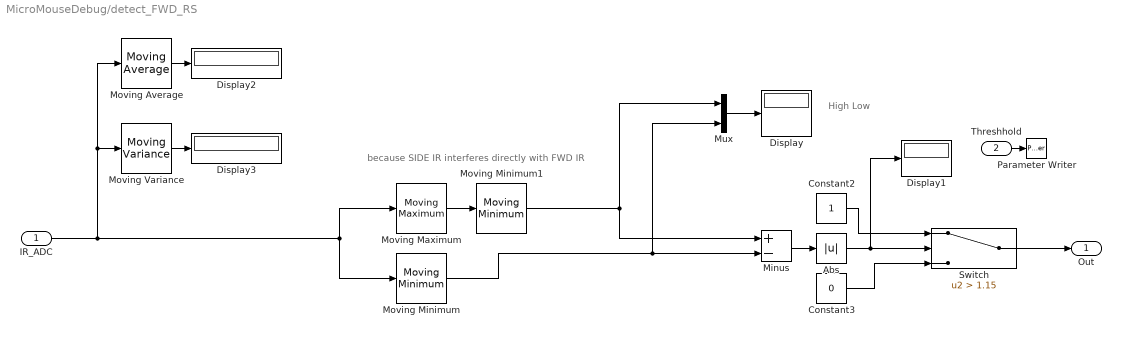
== system MicroMouseDebug/detect_FWD_RS ==
  note: because SIDE IR interferes directly with FWD IR
  note: High
      | Low
  IR_ADC : Inport
  Threshhold : Inport  Port=2
  Abs : Abs  SaturateOnIntegerOverflow=off
  Constant2 : Constant
  Constant3 : Constant  Value=0
  Display{,1..3} (4 alike) : Display
  Minus : Sum  Inputs=+-  AccumDataTypeStr=single  OutDataTypeStr=single
  Moving Average : dspstat3/Moving Average  Method=Sliding window  ForgettingFactorPort=off  SpecifyWindowLength=on  WindowLength=4  OverlapLength=3  AllowArbitraryInputLength=off  ForgettingFactor=0.9  SimulateUsing=Code generation
  Moving Maximum : dspstat3/Moving Maximum  SpecifyWindowLength=on  WindowLength=5  SimulateUsing=Code generation
  Moving Minimum : dspstat3/Moving Minimum  SpecifyWindowLength=on  WindowLength=15  SimulateUsing=Code generation
  Moving Minimum1 : dspstat3/Moving Minimum  SpecifyWindowLength=on  WindowLength=15  SimulateUsing=Code generation
  Moving Variance : dspstat3/Moving Variance  Method=Sliding window  ForgettingFactorPort=off  SpecifyWindowLength=on  WindowLength=4  OverlapLength=3  AllowArbitraryInputLength=off  ForgettingFactor=0.9  SimulateUsing=Code generation
  Mux : Mux  Inputs=2
  Parameter Writer : ParameterWriter  ParameterOwnerBlock=../Switch  ParameterName=Threshold  ParameterInternalName=Threshold
  Switch : Switch  Criteria=u2 > Threshold  Threshold=1.15  SaturateOnIntegerOverflow=off  InputSameDT=off
  Out : Outport
  wires:
  Minus/1 -> Abs/1
  Constant2/1 -> Switch/1
  Moving Minimum/1 -> Minus/2, Mux/2
  Switch/1 -> Out/1
  Constant3/1 -> Switch/3
  Moving Maximum/1 -> Moving Minimum1/1
  Mux/1 -> Display/1
  IR_ADC/1 -> Moving Average/1, Moving Variance/1, Moving Minimum/1, Moving Maximum/1
  Abs/1 -> Switch/2, Display1/1
  Moving Average/1 -> Display2/1
  Moving Variance/1 -> Display3/1
  Threshhold/1 -> Parameter Writer/1
  Moving Minimum1/1 -> Mux/1, Minus/1

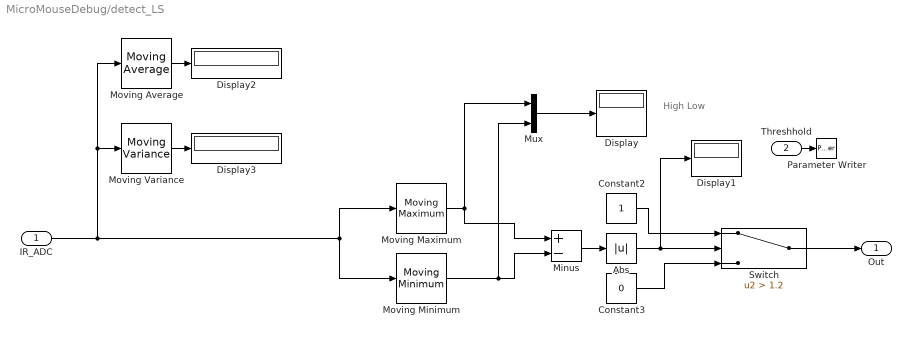
== system MicroMouseDebug/detect_LS ==
  note: High
      | Low
  IR_ADC : Inport
  Threshhold : Inport  Port=2
  Abs : Abs  SaturateOnIntegerOverflow=off
  Constant2 : Constant
  Constant3 : Constant  Value=0
  Display{,1..3} (4 alike) : Display
  Minus : Sum  Inputs=+-  AccumDataTypeStr=single  OutDataTypeStr=single
  Moving Average : dspstat3/Moving Average  Method=Sliding window  ForgettingFactorPort=off  SpecifyWindowLength=on  WindowLength=4  OverlapLength=3  AllowArbitraryInputLength=off  ForgettingFactor=0.9  SimulateUsing=Code generation
  Moving Maximum : dspstat3/Moving Maximum  SpecifyWindowLength=on  WindowLength=15  SimulateUsing=Code generation
  Moving Minimum : dspstat3/Moving Minimum  SpecifyWindowLength=on  WindowLength=15  SimulateUsing=Code generation
  Moving Variance : dspstat3/Moving Variance  Method=Sliding window  ForgettingFactorPort=off  SpecifyWindowLength=on  WindowLength=4  OverlapLength=3  AllowArbitraryInputLength=off  ForgettingFactor=0.9  SimulateUsing=Code generation
  Mux : Mux  Inputs=2
  Parameter Writer : ParameterWriter  ParameterOwnerBlock=../Switch  ParameterName=Threshold  ParameterInternalName=Threshold
  Switch : Switch  Criteria=u2 > Threshold  Threshold=1.2  SaturateOnIntegerOverflow=off  InputSameDT=off
  Out : Outport
  wires:
  Minus/1 -> Abs/1
  Constant2/1 -> Switch/1
  Moving Minimum/1 -> Mux/2, Minus/2
  Switch/1 -> Out/1
  Constant3/1 -> Switch/3
  Moving Maximum/1 -> Mux/1, Minus/1
  Mux/1 -> Display/1
  IR_ADC/1 -> Moving Average/1, Moving Variance/1, Moving Minimum/1, Moving Maximum/1
  Abs/1 -> Switch/2, Display1/1
  Moving Average/1 -> Display2/1
  Moving Variance/1 -> Display3/1
  Threshhold/1 -> Parameter Writer/1

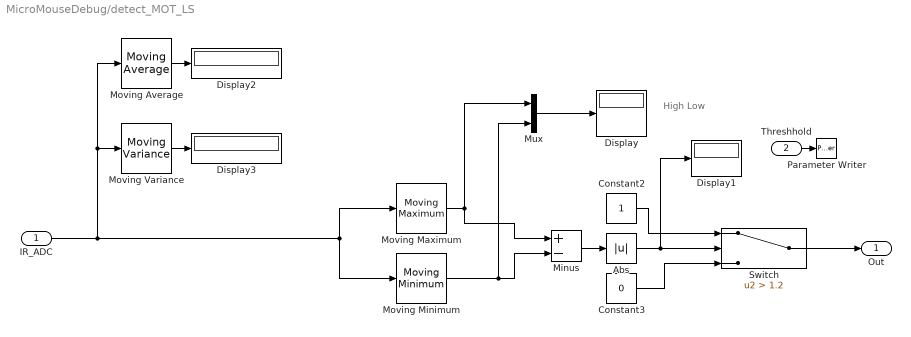
== system MicroMouseDebug/detect_MOT_LS ==
  note: High
      | Low
  IR_ADC : Inport
  Threshhold : Inport  Port=2
  Abs : Abs  SaturateOnIntegerOverflow=off
  Constant2 : Constant
  Constant3 : Constant  Value=0
  Display{,1..3} (4 alike) : Display
  Minus : Sum  Inputs=+-  AccumDataTypeStr=single  OutDataTypeStr=single
  Moving Average : dspstat3/Moving Average  Method=Sliding window  ForgettingFactorPort=off  SpecifyWindowLength=on  WindowLength=4  OverlapLength=3  AllowArbitraryInputLength=off  ForgettingFactor=0.9  SimulateUsing=Code generation
  Moving Maximum : dspstat3/Moving Maximum  SpecifyWindowLength=on  WindowLength=15  SimulateUsing=Code generation
  Moving Minimum : dspstat3/Moving Minimum  SpecifyWindowLength=on  WindowLength=15  SimulateUsing=Code generation
  Moving Variance : dspstat3/Moving Variance  Method=Sliding window  ForgettingFactorPort=off  SpecifyWindowLength=on  WindowLength=4  OverlapLength=3  AllowArbitraryInputLength=off  ForgettingFactor=0.9  SimulateUsing=Code generation
  Mux : Mux  Inputs=2
  Parameter Writer : ParameterWriter  ParameterOwnerBlock=../Switch  ParameterName=Threshold  ParameterInternalName=Threshold
  Switch : Switch  Criteria=u2 > Threshold  Threshold=1.2  SaturateOnIntegerOverflow=off  InputSameDT=off
  Out : Outport
  wires:
  Minus/1 -> Abs/1
  Constant2/1 -> Switch/1
  Moving Minimum/1 -> Mux/2, Minus/2
  Switch/1 -> Out/1
  Constant3/1 -> Switch/3
  Moving Maximum/1 -> Mux/1, Minus/1
  Mux/1 -> Display/1
  IR_ADC/1 -> Moving Average/1, Moving Variance/1, Moving Minimum/1, Moving Maximum/1
  Abs/1 -> Switch/2, Display1/1
  Moving Average/1 -> Display2/1
  Moving Variance/1 -> Display3/1
  Threshhold/1 -> Parameter Writer/1

== system MicroMouseDebug/detect_MOT_RS ==
  note: High
      | Low
  IR_ADC : Inport
  Threshhold : Inport  Port=2
  Abs : Abs  SaturateOnIntegerOverflow=off
  Constant2 : Constant
  Constant3 : Constant  Value=0
  Display{,1..3} (4 alike) : Display
  Minus : Sum  Inputs=+-  AccumDataTypeStr=single  OutDataTypeStr=single
  Moving Average : dspstat3/Moving Average  Method=Sliding window  ForgettingFactorPort=off  SpecifyWindowLength=on  WindowLength=4  OverlapLength=3  AllowArbitraryInputLength=off  ForgettingFactor=0.9  SimulateUsing=Code generation
  Moving Maximum : dspstat3/Moving Maximum  SpecifyWindowLength=on  WindowLength=15  SimulateUsing=Code generation
  Moving Minimum : dspstat3/Moving Minimum  SpecifyWindowLength=on  WindowLength=15  SimulateUsing=Code generation
  Moving Variance : dspstat3/Moving Variance  Method=Sliding window  ForgettingFactorPort=off  SpecifyWindowLength=on  WindowLength=4  OverlapLength=3  AllowArbitraryInputLength=off  ForgettingFactor=0.9  SimulateUsing=Code generation
  Mux : Mux  Inputs=2
  Parameter Writer : ParameterWriter  ParameterOwnerBlock=../Switch  ParameterName=Threshold  ParameterInternalName=Threshold
  Switch : Switch  Criteria=u2 > Threshold  Threshold=1.2  SaturateOnIntegerOverflow=off  InputSameDT=off
  Out : Outport
  wires:
  Minus/1 -> Abs/1
  Constant2/1 -> Switch/1
  Moving Minimum/1 -> Mux/2, Minus/2
  Switch/1 -> Out/1
  Constant3/1 -> Switch/3
  Moving Maximum/1 -> Mux/1, Minus/1
  Mux/1 -> Display/1
  IR_ADC/1 -> Moving Average/1, Moving Variance/1, Moving Minimum/1, Moving Maximum/1
  Abs/1 -> Switch/2, Display1/1
  Moving Average/1 -> Display2/1
  Moving Variance/1 -> Display3/1
  Threshhold/1 -> Parameter Writer/1

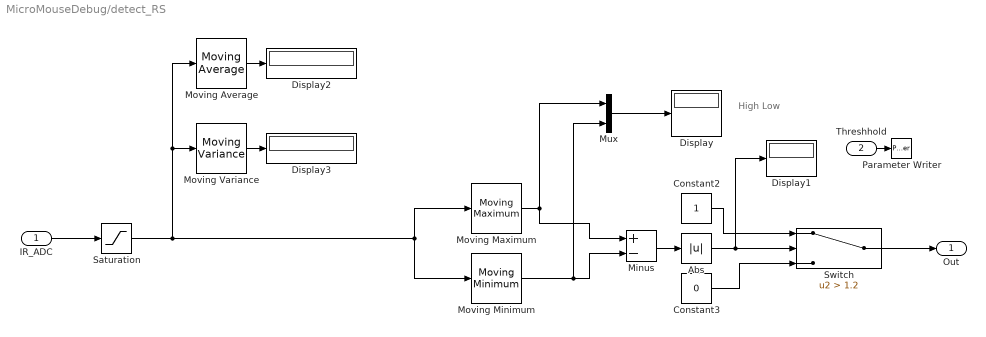
== system MicroMouseDebug/detect_RS ==
  note: High
      | Low
  IR_ADC : Inport
  Threshhold : Inport  Port=2
  Abs : Abs  SaturateOnIntegerOverflow=off
  Constant2 : Constant
  Constant3 : Constant  Value=0
  Display{,1..3} (4 alike) : Display
  Minus : Sum  Inputs=+-  AccumDataTypeStr=single  OutDataTypeStr=single
  Moving Average : dspstat3/Moving Average  Method=Sliding window  ForgettingFactorPort=off  SpecifyWindowLength=on  WindowLength=10  OverlapLength=3  AllowArbitraryInputLength=on  ForgettingFactor=0.9  SimulateUsing=Code generation
  Moving Maximum : dspstat3/Moving Maximum  SpecifyWindowLength=on  WindowLength=15  SimulateUsing=Code generation
  Moving Minimum : dspstat3/Moving Minimum  SpecifyWindowLength=on  WindowLength=15  SimulateUsing=Code generation
  Moving Variance : dspstat3/Moving Variance  Method=Sliding window  ForgettingFactorPort=off  SpecifyWindowLength=on  WindowLength=4  OverlapLength=3  AllowArbitraryInputLength=off  ForgettingFactor=0.9  SimulateUsing=Code generation
  Mux : Mux  Inputs=2
  Parameter Writer : ParameterWriter  ParameterOwnerBlock=../Switch  ParameterName=Threshold  ParameterInternalName=Threshold
  Saturation : Saturate  UpperLimit=3.3  LowerLimit=0
  Switch : Switch  Criteria=u2 > Threshold  Threshold=1.2  SaturateOnIntegerOverflow=off  InputSameDT=off
  Out : Outport
  wires:
  Minus/1 -> Abs/1
  Constant2/1 -> Switch/1
  Moving Minimum/1 -> Mux/2, Minus/2
  Switch/1 -> Out/1
  Constant3/1 -> Switch/3
  Moving Maximum/1 -> Mux/1, Minus/1
  Mux/1 -> Display/1
  IR_ADC/1 -> Saturation/1
  Abs/1 -> Switch/2, Display1/1
  Moving Average/1 -> Display2/1
  Moving Variance/1 -> Display3/1
  Threshhold/1 -> Parameter Writer/1
  Saturation/1 -> Moving Average/1, Moving Variance/1, Moving Minimum/1, Moving Maximum/1

== stateflow chart MicroMouseDebug/Chart ==
  state SuperState
    entry:
    during:
    V_MOT_LS = ADC(1);
    V_FWD_LS = ADC(2);
    V_LS           = ADC(3);
    V_DOWN_LS = ADC(4);
    V_DOWN_RS = ADC(5);
    V_RS           = ADC(6);
    V_FWD_RS = ADC(7);
    V_MOT_RS = ADC(8);
    state Calibrate
      state Cal1
        entry:
        IR_LED_out = [0 0 0 0 0 0 0 0];
        during:
        LED0 = ~LED0;
        LED1 = ~LED1;
        LED2 = ~LED2;
        exit:
        LED0 = false;
        LED1 = false;
        LED2 = false;
      state Cal2
        entry:
        vThreshLower = ADC_H - ADC_L;
      state Cal3
        entry:
        IR_LED_out = IR_LED_in;
      state Cal4
        entry:
        vThreshUpper = ADC_H - ADC_L;
        Thresholds = (vThreshUpper + vThreshLower)/2;
        exit:
        LED0 = true;
        LED1 = true;
        LED2 = true;
      (default) -> Cal1
      Cal1 -> Cal2 : [SW1]
      Cal2 -> Cal3 : [SW2]
      Cal3 -> Cal4 : after(1,sec)
    (default) -> Calibrate
  data: ADC input; V_FWD_LS local; V_FWD_RS local; V_LS local; V_MOT_LS local; V_MOT_RS local; V_RS local; V_DOWN_LS local; V_DOWN_RS local; SW1 input; SW2 input; LED0 output boolean =false; LED1 output boolean =false; LED2 output boolean =false; vThreshLower local; ADC_H input; ADC_L input; IR_LED_out output uint8; Thresholds output; vThreshUpper local; IR_LED_in input
